simulink model "untitled_lamp"  (R2017b)
settings: Solver=VariableStepAuto  StartTime=0.0  StopTime=inf  RelTol=1e-3
settings Model: Creator=Bijan  LastModifiedBy=Bijan

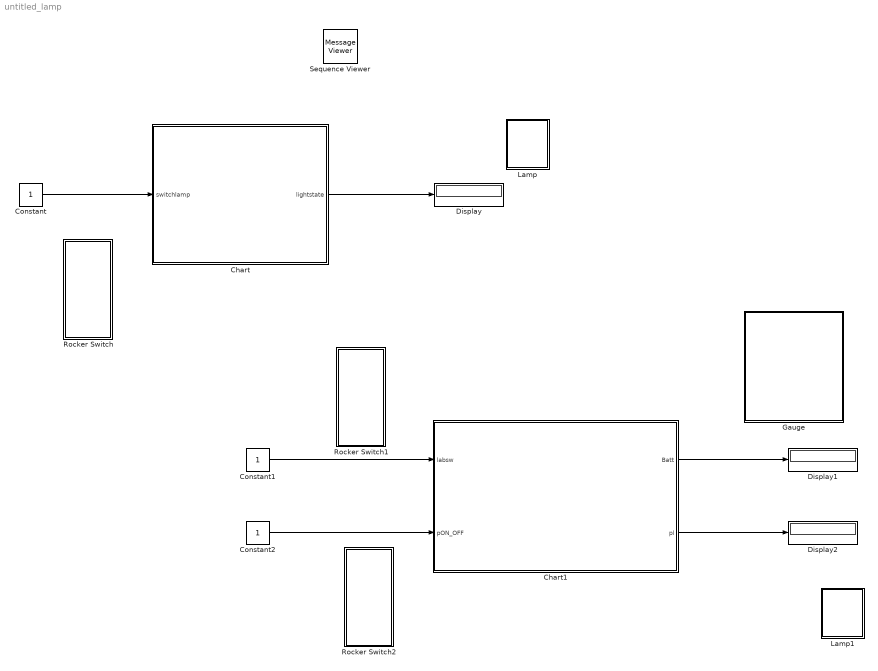
== system untitled_lamp ==
  Chart : Stateflow chart  TreatAsAtomicUnit=on
  Chart1 : Stateflow chart  TreatAsAtomicUnit=on
  Constant : Constant
  Constant1 : Constant
  Constant2 : Constant
  Display : Display
  Display1 : Display
  Display2 : Display
  Gauge : Subsystem  DialogController=hmiCreateDDGDialog  IsWebBlock=on  mask(MWDashboardBlock){webBlockId=c6db0e89-1c08-485c-8588-789685c3c11c, webBlockType=circulargauge, ShowInLibBrowser=on, ShowInitialText=on, HMISrcModelName=untitled_lamp}
      mask prompts: webBlockId "WebBlock Id"; webBlockType "WebBlock Type"; HMISrcModelName "Source Model"
      mask help: SimulinkHMI:dialogs:CircularGaugeDialogDesc
      mask Help: helpview([docroot '/mapfiles/simulink.map'], 'hmi_gauge')
      mask Display:
      | if strcmp(get_param(bdroot(gcb),'BlockDiagramType'), 'library')
      |     image([(matlabroot) '/toolbox/simulink/hmi/icons/CircularGauge.png']);
      | end
  Lamp : Subsystem  DialogController=hmiCreateDDGDialog  IsWebBlock=on  mask(MWDashboardBlock){webBlockId=080a0f5a-9d25-430e-b9d2-b83e69420bc5, webBlockType=lamp, ShowInLibBrowser=on, ShowInitialText=on, HMISrcModelName=untitled_lamp}
      mask prompts: webBlockType "WebBlock Type"; HMISrcModelName "Source Model"
      mask help: SimulinkHMI:dialogs:LampDialogDesc
      mask Help: helpview([docroot '/mapfiles/simulink.map'], 'hmi_lamp')
      mask Display:
      | if strcmp(get_param(bdroot(gcb),'BlockDiagramType'), 'library')
      |     image([(matlabroot) '/toolbox/simulink/hmi/icons/Lamp.png']);
      | end
  Lamp1 : Subsystem  DialogController=hmiCreateDDGDialog  IsWebBlock=on  mask(MWDashboardBlock){webBlockId=fd7aff60-2e9b-4fd9-aa2c-b59668709c3c, webBlockType=lamp, ShowInLibBrowser=on, ShowInitialText=on, HMISrcModelName=untitled_lamp}
      mask prompts: webBlockType "WebBlock Type"; HMISrcModelName "Source Model"
      mask help: SimulinkHMI:dialogs:LampDialogDesc
      mask Help: helpview([docroot '/mapfiles/simulink.map'], 'hmi_lamp')
      mask Display:
      | if strcmp(get_param(bdroot(gcb),'BlockDiagramType'), 'library')
      |     image([(matlabroot) '/toolbox/simulink/hmi/icons/Lamp.png']);
      | end
  Rocker Switch : Subsystem  DialogController=hmiCreateDDGDialog  IsWebBlock=on  mask(MWDashboardBlock){webBlockId=885135b4-82d5-4405-8c88-f31633ecc61b, webBlockType=rockerswitch, ShowInLibBrowser=on, ShowInitialText=on, HMISrcModelName=untitled_lamp}
      mask prompts: webBlockId "WebBlock Id"; webBlockType "WebBlock Type"; HMISrcModelName "Source Model"
      mask help: SimulinkHMI:dialogs:SwitchDialogDesc
      mask Help: helpview([docroot '/mapfiles/simulink.map'], 'hmi_rocker_switch')
      mask Display:
      | if strcmp(get_param(bdroot(gcb),'BlockDiagramType'), 'library')
      |     image([(matlabroot) '/toolbox/simulink/hmi/icons/RockerSwitch.png']);
      | end
  Rocker Switch1 : Subsystem  DialogController=hmiCreateDDGDialog  IsWebBlock=on  mask(MWDashboardBlock){webBlockId=3eaa3620-f343-4e17-a76c-e52d7f4192c0, webBlockType=rockerswitch, ShowInLibBrowser=on, ShowInitialText=on, HMISrcModelName=untitled_lamp}
      mask prompts: webBlockId "WebBlock Id"; webBlockType "WebBlock Type"; HMISrcModelName "Source Model"
      mask help: SimulinkHMI:dialogs:SwitchDialogDesc
      mask Help: helpview([docroot '/mapfiles/simulink.map'], 'hmi_rocker_switch')
      mask Display:
      | if strcmp(get_param(bdroot(gcb),'BlockDiagramType'), 'library')
      |     image([(matlabroot) '/toolbox/simulink/hmi/icons/RockerSwitch.png']);
      | end
  Rocker Switch2 : Subsystem  DialogController=hmiCreateDDGDialog  IsWebBlock=on  mask(MWDashboardBlock){webBlockId=edcf3af7-3a4f-4a5f-9f88-7d3ac32165e8, webBlockType=rockerswitch, ShowInLibBrowser=on, ShowInitialText=on, HMISrcModelName=untitled_lamp}
      mask prompts: webBlockId "WebBlock Id"; webBlockType "WebBlock Type"; HMISrcModelName "Source Model"
      mask help: SimulinkHMI:dialogs:SwitchDialogDesc
      mask Help: helpview([docroot '/mapfiles/simulink.map'], 'hmi_rocker_switch')
      mask Display:
      | if strcmp(get_param(bdroot(gcb),'BlockDiagramType'), 'library')
      |     image([(matlabroot) '/toolbox/simulink/hmi/icons/RockerSwitch.png']);
      | end
  Sequence Viewer : MessageViewer
  wires:
  Constant/1 -> Chart/1(switchlamp)
  Chart/1(lightstate) -> Display/1
  Constant2/1 -> Chart1/2(pON_OFF)
  Constant1/1 -> Chart1/1(labsw)
  Chart1/1(Batt) -> Display1/1
  Chart1/2(pl) -> Display2/1

== system untitled_lamp/Gauge ==

== system untitled_lamp/Lamp ==

== system untitled_lamp/Lamp1 ==

== system untitled_lamp/Rocker Switch ==

== system untitled_lamp/Rocker Switch1 ==

== system untitled_lamp/Rocker Switch2 ==

== stateflow chart untitled_lamp/Chart1 ==
  state plug [parallel]
    settings: executionOrder=1
    state pluged_out1
      entry: pl=0
    state pluged_in
      entry: pl=1
    (default) -> pluged_out1
    pluged_out1 -> pluged_in : [pON_OFF==1]
    pluged_in -> pluged_out1 : [pON_OFF==0]
  state laptop [parallel]
    settings: executionOrder=2
    state laptopOFF
      (default) -> (junction 10) : {Batt=50}
      laptopOFF -> (junction 10) [order 1]
      (junction 10) -> (junction 11) [order 1] : [pl==1]
      (junction 10) -> (junction 15) [order 2] : {Batt=Batt}
      (junction 11) -> (junction 13) : {Batt=Batt+0.001}
      (junction 13) -> (junction 15)
    state laptopON
      (junction 20) -> (junction 21) [order 1] : [pl==0]
      laptopON -> (junction 20) [order 1]
      (junction 21) -> (junction 25) : {Batt=Batt-0.001}
      (junction 20) -> (junction 27) [order 2] : {Batt=Batt+0.001}
      (junction 25) -> (junction 27)
    (default) -> laptopOFF
    laptopOFF -> laptopON [order 1] : [labsw==1]
    laptopON -> laptopOFF [order 1] : [labsw==0]
  data: labsw input; pON_OFF input; Batt output; pl output

== stateflow chart untitled_lamp/Chart ==
  state off
    entry: lightstate=0
  state on
    entry: lightstate=1
  (default) -> off
  off -> on : [switchlamp == 1]
  on -> off : [switchlamp == 0]
  data: lightstate output; switchlamp input
